simulink model "vidu05"  (R2016a)
settings: Solver=VariableStepAuto  StartTime=0.0  StopTime=10.0  RelTol=1e-3
settings Model: Creator=Lenovo  LastModifiedBy=Lenovo

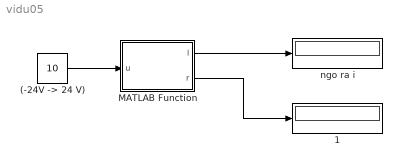
== system vidu05 ==
  "(-24V -> 24 V) " : Constant  Value=10
  1 : Display
  MATLAB Function : MATLAB Function  TreatAsAtomicUnit=on
  "ngo ra i " : Display
  wires:
  "(-24V -> 24 V) "/1 -> MATLAB Function/1(u)
  MATLAB Function/1(l) -> "ngo ra i "/1
  MATLAB Function/2(r) -> 1/1

== matlab function vidu05/MATLAB Function ==
  data: u input; l output; r output
function [l,r] = fcn(u)
%#codegen
    if  u > 0
        r=1;
        l=0;
    elseif u < 0
        r=0;
        l=1;
    else
        r=0;
        l=0;
    end
end
